simulink subsystem "lstm_turboShaftEngineR24a"  (R2024a)
settings: Solver=VariableStepAuto  StartTime=0.0  StopTime=10.0  RelTol=1e-3
undefined symbols (not defined in the file): rom
libraries: deeplib x1
settings Model: Creator=imyrsini  LastModifiedBy=imyrsini
settings RTWCC: GPUComputeCapability=3.5

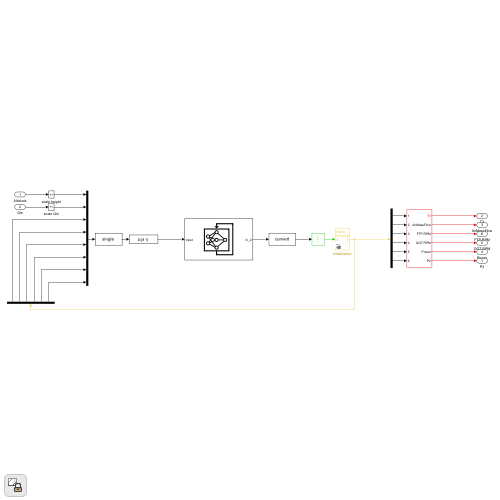
[thumbnail: Simulink's stored preview of the top-level diagram]
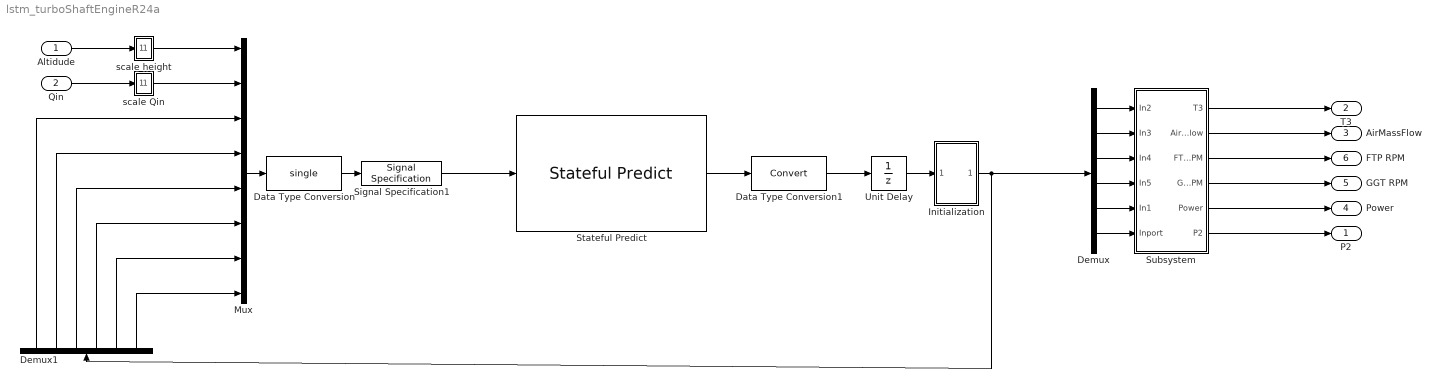
== system lstm_turboShaftEngineR24a ==
  Altidude : Inport
  Qin : Inport  Port=2
  Data Type Conversion : DataTypeConversion  OutDataTypeStr=single  SaturateOnIntegerOverflow=off  RndMeth=Floor
  Data Type Conversion1 : DataTypeConversion  SaturateOnIntegerOverflow=off  RndMeth=Floor
  Demux : Demux  Outputs=6
  Demux1 : Demux  Outputs=6
  Initialization : Subsystem  Variant=on  VariantControlMode=label  VariantControl=Choice  LabelModeActiveChoice=Choice_1
  Mux : Mux  Inputs=8
  Signal Specification1 : SignalSpecification  Dimensions=[8 1]
  Stateful Predict : deeplib/Stateful Predict  Network=Network from MAT-file  NetworkFunction=untitled  NetworkFilePath=C:\Users\imyrsini\OneDrive - MathWorks\Desktop\lstm-model-reduction\SandboxR24a_turboShaftEngine\Models\Components\turboShaftEngineLSTM_ROM\turboshaft_ROM_v5.mat  InputDataFormats={ 'input', 'CBT' }  SampleTime=-1  ForceInterpretedSim=off  EnableDLNetwork=on  LastKnownNetworkFilePath=''  LastKnownNetworkTimeStamp=''
  Subsystem : Subsystem
  Unit Delay : UnitDelay  InitialCondition=[rom.init.AirMassFlow; rom.init.fptRPM; rom.init.ggtRPM; rom.init.power; rom.init.T3; rom.init.p2]  SampleTime=-1  HasFrameUpgradeWarning=on
  scale Qin : Subsystem
  scale height : Subsystem
  P2 : Outport
  T3 : Outport  Port=2
  AirMassFlow : Outport  Port=3
  Power : Outport  Port=4
  GGT RPM : Outport  Port=5
  FTP RPM : Outport  Port=6
  wires:
  Signal Specification1/1 -> Stateful Predict/1
  Mux/1 -> Data Type Conversion/1
  Demux1/6 -> Mux/8
  Stateful Predict/1 -> Data Type Conversion1/1
  Data Type Conversion1/1 -> Unit Delay/1
  Demux1/1 -> Mux/3
  Demux1/5 -> Mux/7
  Demux1/4 -> Mux/6
  Demux1/3 -> Mux/5
  Demux1/2 -> Mux/4
  Qin/1 -> scale Qin/1(In1)
  Altidude/1 -> scale height/1(In1)
  scale height/1(Out1) -> Mux/1
  scale Qin/1(Out1) -> Mux/2
  Subsystem/1(T3) -> T3/1
  Subsystem/2(AirMassFlow) -> AirMassFlow/1
  Subsystem/3(FTP RPM) -> FTP RPM/1
  Subsystem/4(GGT RPM) -> GGT RPM/1
  Subsystem/5(Power) -> Power/1
  Subsystem/6(P2) -> P2/1
  Demux/1 -> Subsystem/1(In2)
  Demux/2 -> Subsystem/2(In3)
  Demux/3 -> Subsystem/3(In4)
  Demux/4 -> Subsystem/4(In5)
  Demux/5 -> Subsystem/5(In1)
  Demux/6 -> Subsystem/6(Inport)
  Unit Delay/1 -> Initialization/1(In1)
  Initialization/1(Out1) -> Demux1/1, Demux/1
  Data Type Conversion/1 -> Signal Specification1/1

== system lstm_turboShaftEngineR24a/Initialization ==
  In1 : Inport
  "Cold Initialization " : Subsystem  VariantControl=Choice
  Warm Initialization : Subsystem  VariantControl=Choice_1
  Out1 : Outport

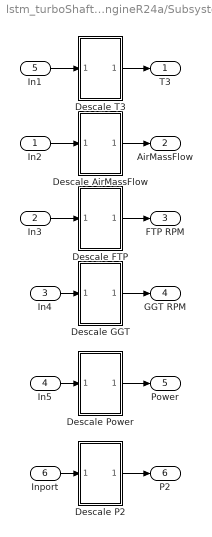
== system lstm_turboShaftEngineR24a/Subsystem ==
  In2 : Inport
  In3 : Inport  Port=2
  In4 : Inport  Port=3
  In5 : Inport  Port=4
  In1 : Inport  Port=5
  Inport : Inport  Port=6
  Descale AirMassFlow : Subsystem
  Descale FTP : Subsystem
  Descale GGT : Subsystem
  Descale P2 : Subsystem
  Descale Power : Subsystem
  Descale T3 : Subsystem
  T3 : Outport
  AirMassFlow : Outport  Port=2
  FTP RPM : Outport  Port=3
  GGT RPM : Outport  Port=4
  Power : Outport  Port=5
  P2 : Outport  Port=6
  wires:
  Descale P2/1(Out1) -> P2/1
  Inport/1 -> Descale P2/1(In1)
  In5/1 -> Descale Power/1(In1)
  In4/1 -> Descale GGT/1(In1)
  Descale T3/1(Out1) -> T3/1
  In2/1 -> Descale AirMassFlow/1(In1)
  In3/1 -> Descale FTP/1(In1)
  In1/1 -> Descale T3/1(In1)
  Descale Power/1(Out1) -> Power/1
  Descale FTP/1(Out1) -> FTP RPM/1
  Descale AirMassFlow/1(Out1) -> AirMassFlow/1
  Descale GGT/1(Out1) -> GGT RPM/1

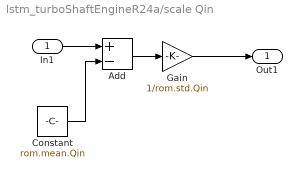
== system lstm_turboShaftEngineR24a/scale Qin ==
  In1 : Inport
  Add : Sum  Inputs=+-
  Constant : Constant  Value=rom.mean.Qin
  Gain : Gain  Gain=1/rom.std.Qin
  Out1 : Outport
  wires:
  In1/1 -> Add/1
  Constant/1 -> Add/2
  Add/1 -> Gain/1
  Gain/1 -> Out1/1

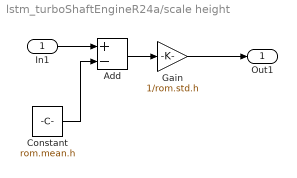
== system lstm_turboShaftEngineR24a/scale height ==
  In1 : Inport
  Add : Sum  Inputs=+-
  Constant : Constant  Value=rom.mean.h
  Gain : Gain  Gain=1/rom.std.h
  Out1 : Outport
  wires:
  Gain/1 -> Out1/1
  Add/1 -> Gain/1
  Constant/1 -> Add/2
  In1/1 -> Add/1

== system lstm_turboShaftEngineR24a/Initialization/Cold Initialization  ==
  In1 : Inport
  Out1 : Outport
  wires:
  In1/1 -> Out1/1

== system lstm_turboShaftEngineR24a/Initialization/Warm Initialization ==
  In1 : Inport
  Warm Initialization : Subsystem  VariantControl=Choice
  Out1 : Outport
  wires:
  In1/1 -> Warm Initialization/1(In1)
  Warm Initialization/1(Out1) -> Out1/1

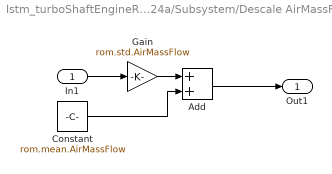
== system lstm_turboShaftEngineR24a/Subsystem/Descale AirMassFlow ==
  In1 : Inport
  Add : Sum
  Constant : Constant  Value=rom.mean.AirMassFlow
  Gain : Gain  Gain=rom.std.AirMassFlow
  Out1 : Outport
  wires:
  In1/1 -> Gain/1
  Add/1 -> Out1/1
  Gain/1 -> Add/1
  Constant/1 -> Add/2

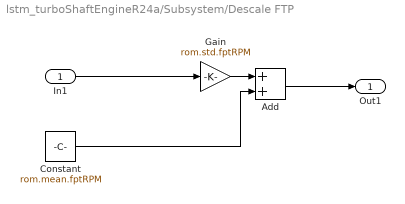
== system lstm_turboShaftEngineR24a/Subsystem/Descale FTP ==
  In1 : Inport
  Add : Sum
  Constant : Constant  Value=rom.mean.fptRPM
  Gain : Gain  Gain=rom.std.fptRPM
  Out1 : Outport
  wires:
  In1/1 -> Gain/1
  Constant/1 -> Add/2
  Gain/1 -> Add/1
  Add/1 -> Out1/1

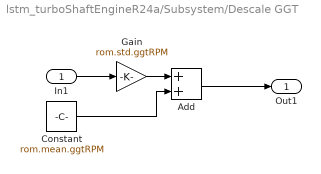
== system lstm_turboShaftEngineR24a/Subsystem/Descale GGT ==
  In1 : Inport
  Add : Sum
  Constant : Constant  Value=rom.mean.ggtRPM
  Gain : Gain  Gain=rom.std.ggtRPM
  Out1 : Outport
  wires:
  In1/1 -> Gain/1
  Add/1 -> Out1/1
  Gain/1 -> Add/1
  Constant/1 -> Add/2

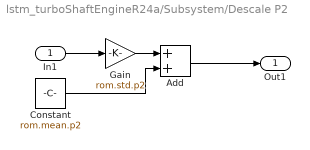
== system lstm_turboShaftEngineR24a/Subsystem/Descale P2 ==
  In1 : Inport
  Add : Sum
  Constant : Constant  Value=rom.mean.p2
  Gain : Gain  Gain=rom.std.p2
  Out1 : Outport
  wires:
  In1/1 -> Gain/1
  Add/1 -> Out1/1
  Gain/1 -> Add/1
  Constant/1 -> Add/2

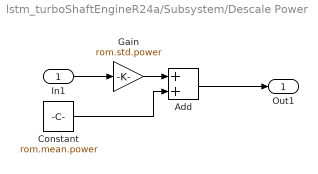
== system lstm_turboShaftEngineR24a/Subsystem/Descale Power ==
  In1 : Inport
  Add : Sum
  Constant : Constant  Value=rom.mean.power
  Gain : Gain  Gain=rom.std.power
  Out1 : Outport
  wires:
  Constant/1 -> Add/2
  Gain/1 -> Add/1
  Add/1 -> Out1/1
  In1/1 -> Gain/1

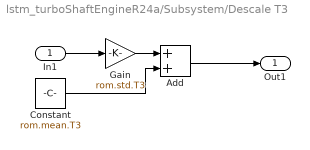
== system lstm_turboShaftEngineR24a/Subsystem/Descale T3 ==
  In1 : Inport
  Add : Sum
  Constant : Constant  Value=rom.mean.T3
  Gain : Gain  Gain=rom.std.T3
  Out1 : Outport
  wires:
  Constant/1 -> Add/2
  Gain/1 -> Add/1
  Add/1 -> Out1/1
  In1/1 -> Gain/1

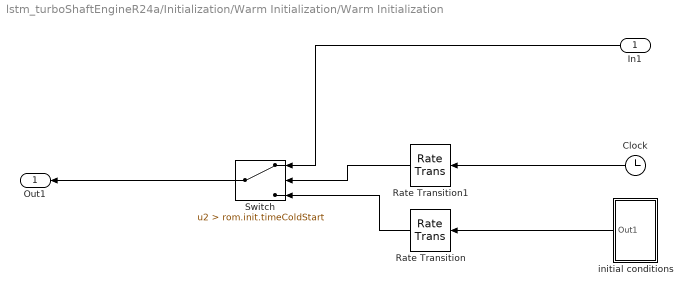
== system lstm_turboShaftEngineR24a/Initialization/Warm Initialization/Warm Initialization ==
  In1 : Inport
  Clock : Clock
  Rate Transition : RateTransition  Integrity=off  OutPortSampleTime=sampleTime
  Rate Transition1 : RateTransition  Integrity=off  OutPortSampleTime=sampleTime
  Switch : Switch  Criteria=u2 > Threshold  Threshold=rom.init.timeColdStart  SaturateOnIntegerOverflow=off  InputSameDT=off
  initial conditions : Subsystem
  Out1 : Outport
  wires:
  Rate Transition1/1 -> Switch/2
  Switch/1 -> Out1/1
  In1/1 -> Switch/1
  Clock/1 -> Rate Transition1/1
  Rate Transition/1 -> Switch/3
  initial conditions/1(Out1) -> Rate Transition/1

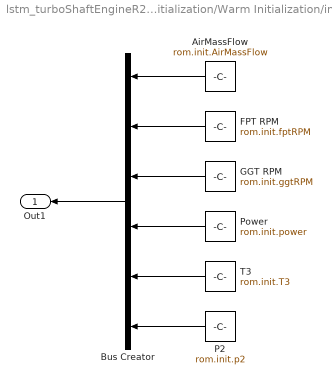
== system lstm_turboShaftEngineR24a/Initialization/Warm Initialization/Warm Initialization/initial conditions ==
  AirMassFlow : Constant  Value=rom.init.AirMassFlow
  Bus Creator : BusCreator  Inputs=6
  FPT RPM : Constant  Value=rom.init.fptRPM
  GGT RPM : Constant  Value=rom.init.ggtRPM
  P2 : Constant  Value=rom.init.p2
  Power : Constant  Value=rom.init.power
  T3 : Constant  Value=rom.init.T3
  Out1 : Outport
  wires:
  Bus Creator/1 -> Out1/1
  P2/1 -> Bus Creator/6
  T3/1 -> Bus Creator/5
  Power/1 -> Bus Creator/4
  GGT RPM/1 -> Bus Creator/3
  FPT RPM/1 -> Bus Creator/2
  AirMassFlow/1 -> Bus Creator/1
